simulink model "control_scheme"  (R2023b)
settings: Solver=VariableStepAuto  StartTime=0.0  StopTime=50.0  RelTol=1e-3
libraries: instrumentlib x2
settings Model: Creator=pc  LastModifiedBy=pc

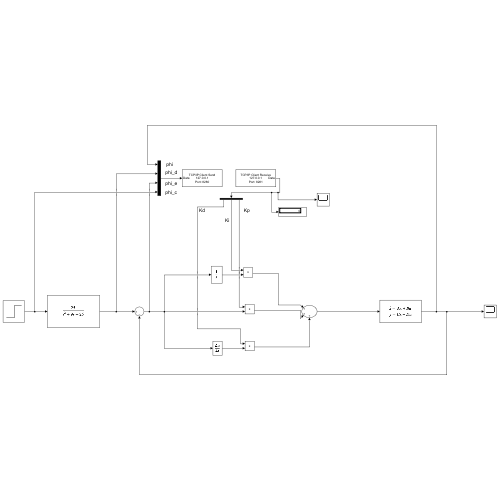
[thumbnail: Simulink's stored preview of the top-level diagram]
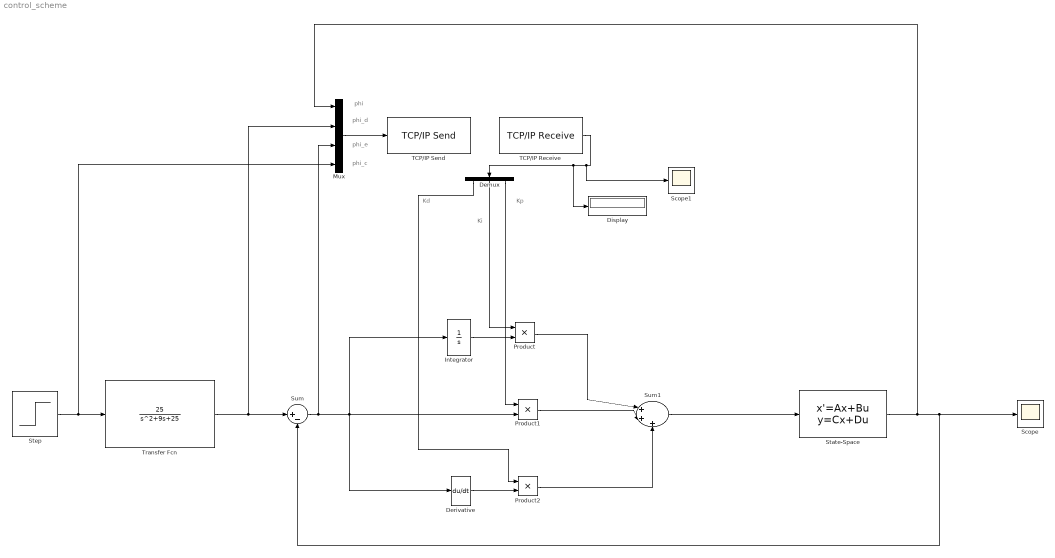
== system control_scheme ==
  note: Ki
  note: Kd
  note: Kp
  note: phi_c
  note: phi_d
  note: phi_e
  note: phi
  Demux : Demux  Outputs=3
  Derivative : Derivative
  Display : Display
  Integrator : Integrator
  Mux : Mux
  Product : Product
  Product1 : Product
  Product2 : Product
  Scope : Scope
  Scope1 : Scope
  State-Space : StateSpace  D=0  InitialCondition=0  ContinuousStateAttributes='Controlled_Object'
  Step : Step  Time=0  Before=1  After=5  SampleTime=0
  Sum : Sum  Inputs=|+-
  Sum1 : Sum  Inputs=|+++
  TCP/IP Receive : instrumentlib/TCP//IP Receive  Host=127.0.0.1  Port=8281  DataSize=[ 3, 1 ]  DataType=double  ASCIIFormatting=%f  Terminator=LF  CustomTerminator=10  ByteOrder=big-endian  EnableBlockingMode=on  Timeout=10  SampleTime=0.01  SimulateUsing=Interpreted execution
  TCP/IP Send : instrumentlib/TCP//IP Send  Host=127.0.0.1  Port=8280  ByteOrder=big-endian  EnableBlockingMode=on  Timeout=10  TransferDelay=on  SimulateUsing=Interpreted execution
  Transfer Fcn : TransferFcn  Numerator=[25]  Denominator=[1 9 25]  ContinuousStateAttributes='Reference_Model'
  wires:
  Step/1 -> Mux/4, Transfer Fcn/1
  Transfer Fcn/1 -> Mux/2, Sum/1
  State-Space/1 -> Mux/1, Sum/2, Scope/1
  Sum/1 -> Product1/2, Derivative/1, Integrator/1, Mux/3
  Sum1/1 -> State-Space/1
  Mux/1 -> TCP/IP Send/1
  TCP/IP Receive/1 -> Scope1/1, Display/1, Demux/1
  Product1/1 -> Sum1/2
  Product/1 -> Sum1/1
  Product2/1 -> Sum1/3
  Derivative/1 -> Product2/2
  Integrator/1 -> Product/2
  Demux/3 -> Product1/1
  Demux/2 -> Product/1
  Demux/1 -> Product2/1
